simulink model "P3"  (R2019b)
settings: Solver=FixedStepAuto  StartTime=0.0  StopTime=15  FixedStep=1e-3  RelTol=1e-3
values from neighbouring files (symbols this model uses):
  x2_0 = 2.*rand(1,1)-1    [p1_initialization.m]    (also in p3_initialization.m; p4_initialization.m = -1)
  x3_0 = 2.*rand(1,1)-1    [p1_initialization.m]    (also in p3_initialization.m; p4_initialization.m = 3)
  x4_0 = 2.*rand(1,1)-1    [p1_initialization.m]    (also in p3_initialization.m; p4_initialization.m = 1)
settings Model: Creator=cz  LastModifiedBy=cz

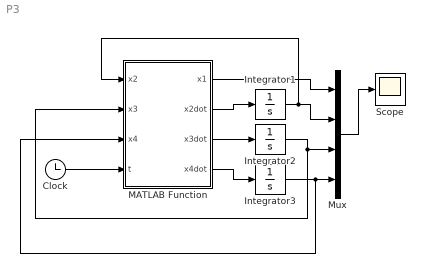
== system P3 ==
  Clock : Clock
  Integrator1 : Integrator  InitialCondition=x2_0
  Integrator2 : Integrator  InitialCondition=x3_0
  Integrator3 : Integrator  InitialCondition=x4_0
  MATLAB Function : MATLAB Function  TreatAsAtomicUnit=on
  Mux : Mux
  Scope : Scope
  wires:
  Clock/1 -> MATLAB Function/4(t)
  MATLAB Function/4(x4dot) -> Integrator3/1
  MATLAB Function/3(x3dot) -> Integrator2/1
  MATLAB Function/2(x2dot) -> Integrator1/1
  MATLAB Function/1(x1) -> Mux/1
  Integrator1/1 -> MATLAB Function/1(x2), Mux/2
  Integrator2/1 -> MATLAB Function/2(x3), Mux/3
  Integrator3/1 -> MATLAB Function/3(x4), Mux/4
  Mux/1 -> Scope/1

== matlab function P3/MATLAB Function ==
  data: x2 input; x1 output; x3 input; x4 input; t input; x2dot output; x3dot output; x4dot output
function [x1,x2dot,x3dot,x4dot] = fcn(x2,x3,x4,t)
k=10;
% x1=0;
% x1=0.1;
x1=0.1*sin(2*t);
% x1=0.5*sin(2*t);
% x1=0.5*sin(0.2*t);
% x1dot=diff(x1,t);
x2dot=k*(x1-x2);
x3dot=k*(x1-x3)+k*(x2-x3);
x4dot=k*(x3-x4);
